simulink model "Motor3Terry"  (Simulink 8.7)
settings: Solver=ode23t  StartTime=0.0  StopTime=10  RelTol=1e-3
PreLoadFcn:
  | Fc = 0.1;
  | Fb = 1;
  | Ts = 0.1;
  | if ~exist('F','var')
  |   load('initialParameters.mat')
  | end
undefined symbols (not defined in the file): sigbuilder_block
libraries: demoLibrary x1, simulink x1
settings Model: Creator=deastman  LastModifiedBy=tdenery
settings DataIOCC: LimitDataPoints=off  SaveOutput=off  SaveTime=off
settings OptimizationCC: ExpressionDepthLimit=2147483647
settings DebuggingCC: FcnCallInpInsideContextMsg=UseLocalSettings  StateNameClashWarn=warning
settings GRTTargetCC: CombineOutputUpdateFcns=off  GRTInterface=on
settings ConfigComp: CovSFcnEnable=off
settings ConfigurationSet: Description=SimMechanics 2G

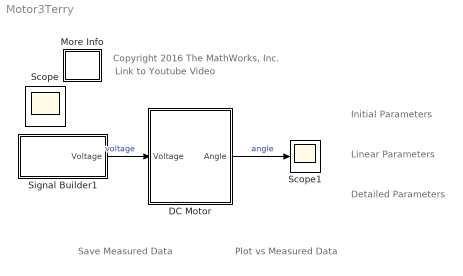
== system Motor3Terry ==
  note: Save Measured Data
  note: Plot vs Measured Data
  note: Initial
      | Parameters
  note: Detailed
      | Parameters
  note: Linear
      | Parameters
  note: Link to Youtube Video
  note: Copyright 2016 The MathWorks, Inc.
  DC Motor : Subsystem  BlockChoice=Open Loop Interface
      link override Open Loop Interface/Serial Motor Interface/Serial Configuration: ComPortMenu=COM4  StopBits=1  ComPort=COM4  ObjConstructor=serial('COM4');
      settings: AttributesFormatString=%<BlockChoice>  TemplateBlock=demoLibrary/Motor Models/DC Motor  MemberBlocks=Detailed Model,Open Loop Interface,SimElectronics Model,SimMechanics w/ Camera,Simple Model,Simscape Model,Simulink Model,Simulink Model with Friction,State Space Model,xPC Target Interface
  More Info : Subsystem
      mask Display: disp('?')
  Scope1 : Scope
  Signal Builder1 : Subsystem  Tag=STV Subsys  LoadFcn=sigbuilder_block('load');  StartFcn=sigbuilder_block('start');  StopFcn=sigbuilder_block('stop');  ClipboardFcn=sigbuilder_block('clipboard');  mask(Sigbuilder block){}
      mask help: Sigbuilder GUI
      mask init:
      | if ~strcmp(get_param(bdroot(gcbh),'SimulationStatus'),'stopped') tuvar = sigbuilder_block('maskInit'); end
      settings: CopyFcn=sigbuilder_block('copy');  DeleteFcn=sigbuilder_block('delete');  ModelCloseFcn=sigbuilder_block('modelClose');  PreSaveFcn=sigbuilder_block('preSave');  PauseFcn=sigbuilder_block('pause')  ContinueFcn=sigbuilder_block('continue')  NameChangeFcn=sigbuilder_block('namechange');  OpenFcn=sigbuilder_block('open',[183.75 96 550.5 399.75 ]);  CloseFcn=sigbuilder_block('close');
      mask Display: plot(0,0,100,100,[10,10,40,40,10],[80,20,20,80,80],[40,10],[50,50], [40,27,10],[65,72,56],[40,25,25,10],[28,28,43,43]);
  Scope : Scope
  wires:
  DC Motor/1(Angle) -> Scope1/1  "angle"
  Signal Builder1/1(Voltage) -> DC Motor/1(Voltage)  "voltage"

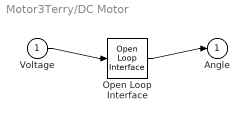
== system Motor3Terry/DC Motor ==
  Voltage : Inport
  Open Loop Interface : demoLibrary/Motor Models/Open Loop Interface  SystemSampleTime=-1
  Angle : Outport
  wires:
  Voltage/1 -> Open Loop Interface/1
  Open Loop Interface/1 -> Angle/1

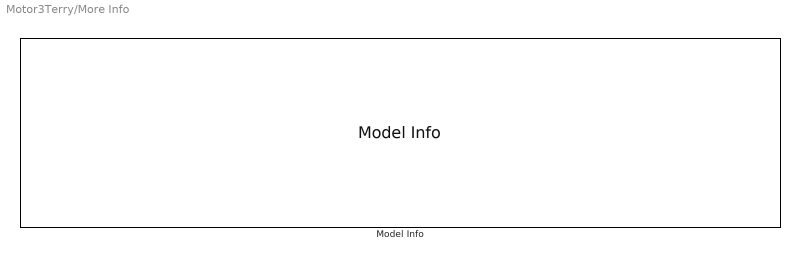
== system Motor3Terry/More Info ==
  Model Info : simulink/Model-Wide Utilities/Model Info  Frame=on  DisplayStringWithTags=|  HorizontalTextAlignment=Left  LeftAlignmentValue=0.02  SourceBlockDiagram=Motor3Terry  TagMaxNumber=20
      | Model Description:
      | -------------------
      | 
      | Robotic Arm Model that is used in the Youtube Video , Mechatronic Systems with MATLAB & Simulink, Part 2:  Importing Mechanics from CAD Tools
      | 
      | https://www.youtube.com/watch?v=w7lAlzgf6UM&index=4&list=PLn8PRpmsu08qFTItUTfJYklhQDEbBpoLt
      | %<Description>

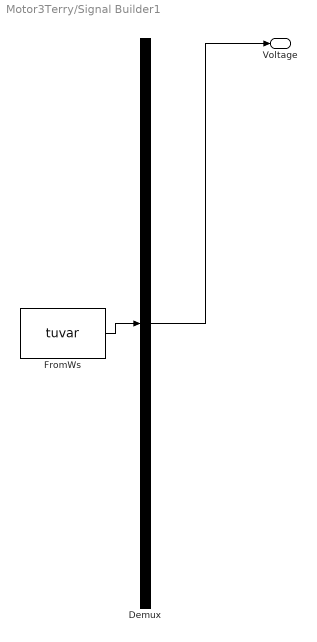
== system Motor3Terry/Signal Builder1 ==
  Demux : Demux  Tag=STV Demux  Outputs=1
  FromWs : FromWorkspace  Tag=STV FromWs  VariableName=tuvar  SampleTime=1/100  SigBuilderData=DataTag0  VnvData=DataTag1
      SigBuilderData=|
      | common.afterFinalStr = 'Extrapolate'
      | common.sampleTime = '1/100'
      | dataSet(1).timeRange = [0 10]
      | dataSet(1).name = 'Bounds'
      | dataSet(2).timeRange = [0 10]
      | dataSet(2).name = 'Steps'
      | dataSet(3).timeRange = [0 10]
      | dataSet(3).name = 'Small Steps'
      | dataSet(4).timeRange = [0 10]
      | dataSet(4).name = 'Square Waves'
      | dataSet(5).timeRange = [0 10]
      | dataSet(5).name = 'Square Waves1'
      | sbobj.Groups(1).Name = 'Bounds'
      | sbobj.Groups(1).Signals.Name = 'Voltage'
      | sbobj.Groups(1).Signals.XData = [0 2 2 2.5 2.5 4.5 4.5 10]
      | sbobj.Groups(1).Signals.YData = [0 0 5 5 0 0 -5 -5]
      | sbobj.Groups(2).Name = 'Steps'
      | sbobj.Groups(2).Signals.Name = 'Voltage'
      | sbobj.Groups(2).Signals.XData = [0 1.52 1.52 2.4 2.4 3.66 3.68 4.64 4.64 6.02 6.02 7 7 8.96 8.96 10]
      | sbobj.Groups(2).Signals.YData = [2 2 -3 -3 3 -1 1.95 1.95 -2 -2 0.7 0.7 -1.05 -0.05 0 0]
      | sbobj.Groups(3).Name = 'Small Steps'
      | sbobj.Groups(3).Signals.Name = 'Voltage'
      | sbobj.Groups(3).Signals.XData = [0 0.5 0.5 1.02 1.02 2 2 2.58 2.58 3.78 3.78 4.64 4.64 5.28 5.28 6 6 7 7 9 9 10]
      | sbobj.Groups(3).Signals.YData = [0.4 0.4 0.75 0.75 1.5 3 1.55 1.55 3.55 3.55 -3.05 -3.05 -1 -1 -0.45 -0.45 0.7 0.7 -2.05 -0.05 1 1]
      | sbobj.Groups(4).Name = 'Square Waves'
      | sbobj.Groups(4).Signals.Name = 'Voltage'
      | sbobj.Groups(4).Signals.XData = [0 0.5 0.5 1.02 1.02 1.5 1.5 2 2 2.5 2.5 3 3 4 4 5 5 6 6 7 7 8 8 9 9 9.8 9.8 10]
      | sbobj.Groups(4).Signals.YData = [0.4 0.4 -0.4 -0.4 1 1 -1 -1 1.5 1.5 -1.5 -1.5 2 2 -2 -2 3 3 -3 -3 1.3 1.3 -1.3 -1.3 -4 -4 0 0]
      | sbobj.Groups(5).Name = 'Square Waves1'
      | sbobj.Groups(5).Signals.Name = 'Voltage'
      | sbobj.Groups(5).Signals.XData = [0 1 1 2 2 3 3 4 4 5 5 6 6 7 7 8 8 9 9 9.8 9.8 10]
      | sbobj.Groups(5).Signals.YData = [0 0.75 0 -0.75 0 1.5 0 -1.5 2 2 -2 -2 3 3 -3 -3 1 1 -1 -1 0 0]
  Voltage : Outport  Tag=STV Outport
  wires:
  Demux/1 -> Voltage/1
  FromWs/1 -> Demux/1
